simulink model "PID_Controller_try1"  (R2024b)
settings: Solver=VariableStepAuto  StartTime=0.0  StopTime=10.0  RelTol=1e-3
undefined symbols (not defined in the file): gaussian
libraries: simulink x1
settings Model: Creator=SURYA  LastModifiedBy=SURYA

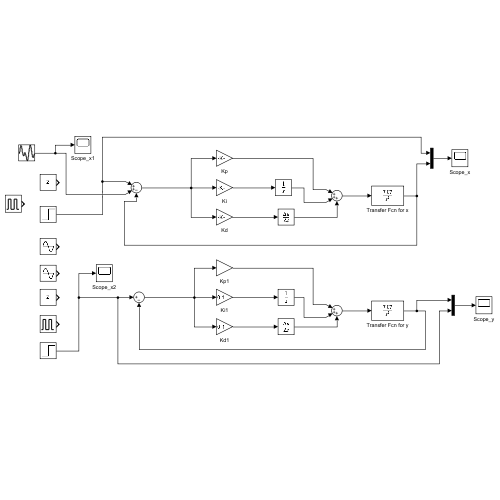
[thumbnail: Simulink's stored preview of the top-level diagram]
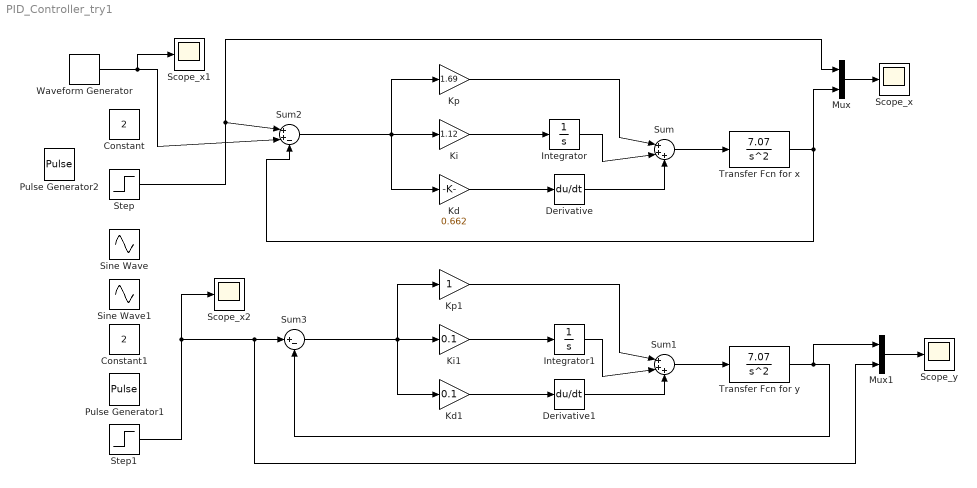
== system PID_Controller_try1 ==
  Constant : Constant  Value=2
  Constant1 : Constant  Value=2
  Derivative : Derivative
  Derivative1 : Derivative
  Integrator : Integrator
  Integrator1 : Integrator
  Kd : Gain  Gain=0.662
  Kd1 : Gain  Gain=0.1
  Ki : Gain  Gain=1.12
  Ki1 : Gain  Gain=0.1
  Kp : Gain  Gain=1.69
  Kp1 : Gain
  Mux : Mux  Inputs=2
  Mux1 : Mux  Inputs=2
  Pulse Generator1 : DiscretePulseGenerator  PulseType=Time based  Period=10  PulseWidth=5
  Pulse Generator2 : DiscretePulseGenerator  PulseType=Time based  Period=10  PulseWidth=5
  Scope_x : Scope
  Scope_x1 : Scope
  Scope_x2 : Scope
  Scope_y : Scope
  Sine Wave : Sin  Frequency=0.5  SampleTime=0
  Sine Wave1 : Sin  Frequency=0.5  SampleTime=0
  Step : Step  SampleTime=0
  Step1 : Step  SampleTime=0
  Sum : Sum  Inputs=|+++
  Sum1 : Sum  Inputs=|+++
  Sum2 : Sum  Inputs=|++-
  Sum3 : Sum  Inputs=|+-
  Transfer Fcn for x : TransferFcn  Numerator=[7.07]  Denominator=[1 0 0]
  Transfer Fcn for y : TransferFcn  Numerator=[7.07]  Denominator=[1 0 0]
  Waveform Generator : simulink/Sources/Waveform Generator  OutMin=[]  OutMax=[]  OutDataTypeStr=double  SelectedSignal=1  Signals=gaussian('Mean', 0, 'Variance', 0.005, 'Seed', 0)  BlockNames=MultiportSwitch_0c18acc982a94b1  SampleTime=0.1
  wires:
  Kp/1 -> Sum/1
  Ki/1 -> Integrator/1
  Kd/1 -> Derivative/1
  Derivative/1 -> Sum/3
  Integrator/1 -> Sum/2
  Sum/1 -> Transfer Fcn for x/1
  Kd1/1 -> Derivative1/1
  Kp1/1 -> Sum1/1
  Ki1/1 -> Integrator1/1
  Integrator1/1 -> Sum1/2
  Sum1/1 -> Transfer Fcn for y/1
  Derivative1/1 -> Sum1/3
  Transfer Fcn for y/1 -> Mux1/1, Sum3/2
  Sum2/1 -> Kp/1, Ki/1, Kd/1
  Sum3/1 -> Kd1/1, Ki1/1, Kp1/1
  Step1/1 -> Scope_x2/1, Mux1/2, Sum3/1
  Mux/1 -> Scope_x/1
  Transfer Fcn for x/1 -> Sum2/3, Mux/2
  Step/1 -> Mux/1, Sum2/1
  Mux1/1 -> Scope_y/1
  Waveform Generator/1 -> Sum2/2, Scope_x1/1
